simulink model "elevator"  (R2024b)
settings: Solver=VariableStepAuto  StartTime=0.0  StopTime=10.0  RelTol=1e-3
settings Model: Creator=Krishna K S  LastModifiedBy=Krishna K S

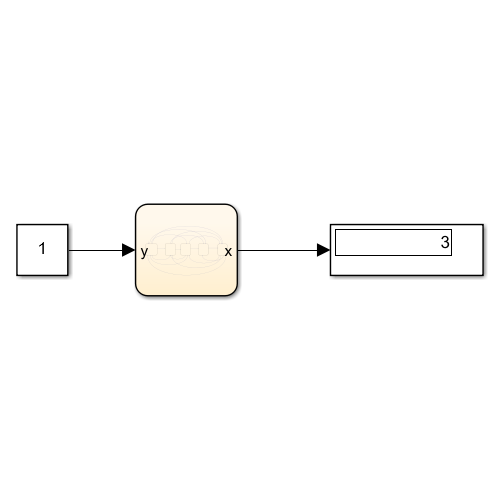
[thumbnail: Simulink's stored preview of the top-level diagram]
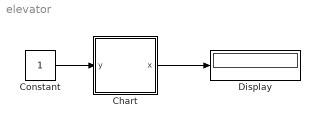
== system elevator ==
  Chart : Stateflow chart  TreatAsAtomicUnit=on
  Constant : Constant
  Display : Display
  wires:
  Chart/1(x) -> Display/1
  Constant/1 -> Chart/1(y)

== stateflow chart elevator/Chart ==
  state F_0
    x=0;
  state F_1
    x=1;
  state F_2
    x=2;
  state F_3
    x=3;
  state F_4
    x=4;
  F_0 -> F_4 [order 4] : [y==4]{after(40,sec)}
  F_0 -> F_3 [order 2] : [y==3]{after(40,sec)}
  F_1 -> F_4 [order 4] : [y==4]{after(40,sec)}
  F_0 -> F_2 [order 3] : [y==2]{after(40,sec)}
  F_1 -> F_3 [order 3] : [y==3]{after(40,sec)}
  F_2 -> F_4 [order 4] : [y==4]{after(40,sec)}
  F_1 -> F_2 [order 5] : [y==3]{after(40,sec)}
  (default) -> F_0
  F_3 -> F_4 : [y==4]{after(40,sec)}
  F_0 -> F_1 [order 1] : [y==1]{after(10,sec)}
  F_2 -> F_3 [order 1] : [y==3]{after(40,sec)}
  F_1 -> F_2 [order 1] : [y==2]{after(10,sec)}
  F_4 -> F_0 [order 1] : [y==0]{after(40,sec)}
  F_2 -> F_0 [order 2] : [y==0]{after(40,sec)}
  F_0 -> F_3 [order 5] : [y==3]{after(40,sec)}
  F_1 -> F_0 [order 2] : [y==0]{after(40,sec)}
  F_2 -> F_1 [order 3] : [y==1]{after(40,sec)}
  F_4 -> F_1 [order 2] : [y==1]{after(40,sec)}
  F_4 -> F_2 [order 3] : [y==2]{after(40,sec)}
  F_4 -> F_3 [order 4] : [y==3]{after(40,sec)}
  data: y input; x output
